simulink model "sim_2_twolink_joint_control_real"  (R2021a)
settings: Solver=ode45  StartTime=0.0  StopTime=15  MaxStep=0.01  RelTol=1e-5  EnableMultiTasking=on
values from neighbouring files (symbols this model uses):
  b1 = 0.01    [sim_params.m]    (also in sim_params_force.m)
  b2 = 0.01    [sim_params.m]    (also in sim_params_force.m)
  D = [zeros(n); eye(n)]    [control_comparison_script.m]    (also in gen_twolink_ss.m = reshape([0.0,0.0,0.0,0.0,0.0,0.0,0.0,0.0],[4,2]))
  D_T_Q = D'*Q    [control_comparison_script.m]
  epsilon = 0.1    [control_comparison_script.m]
  g = 9.80665    [sim_params.m]    (also in sim_params_force.m)
  joint_acc_variance = 0    [sim_params.m]    (also in sim_params_force.m)
  joint_pos_variance = joint_pos_precision^2    (= 0.0001)    [control_comparison_script.m]    (also in sim_params.m = 2.5e-05; sim_params_force.m = 2.5e-05)
  joint_vel_variance = 0    [sim_params.m]    (also in sim_params_force.m)
  Kd1 = 2.5    [control_comparison_script.m]
  Kd1_grav = 2.5    [control_comparison_script.m]
  Kd1_inv = 12    [control_comparison_script.m]
  Kd1_robust = 7    [control_comparison_script.m]
  Kd2 = 0.5    [control_comparison_script.m]
  Kd2_grav = 0.5    [control_comparison_script.m]
  Kd2_inv = 15    [control_comparison_script.m]
  Kd2_robust = 35    [control_comparison_script.m]
  Ki1 = 20    [control_comparison_script.m]
  Ki2 = 15    [control_comparison_script.m]
  Klqr = lqr(A,B,Q,R)    [control_comparison_script.m]
  Kp1 = 30    [control_comparison_script.m]
  Kp1_grav = 15    [control_comparison_script.m]
  Kp1_inv = 25    [control_comparison_script.m]
  Kp1_robust = 25    [control_comparison_script.m]
  Kp2 = 7    [control_comparison_script.m]
  Kp2_grav = 3.5    [control_comparison_script.m]
  Kp2_inv = 50    [control_comparison_script.m]
  Kp2_robust = 45    [control_comparison_script.m]
  Kpp = place(A,B,p)    [control_comparison_script.m]
  L1x = 0.3    [sim_params.m]    (also in sim_params_force.m)
  L1y = 0.050    (= 0.05)    [sim_params.m]    (also in sim_params_force.m)
  L1z = 0.05    [sim_params.m]    (also in sim_params_force.m)
  L2x = 0.15    [sim_params.m]    (also in sim_params_force.m = 0.3)
  L2y = 0.05    [sim_params.m]    (also in sim_params_force.m)
  L2z = 0.05    [sim_params.m]    (also in sim_params_force.m)
  length_dev = (100+randi([-param_dev,param_dev],1))/100.0    [control_comparison_script.m]
  m1 = m1*1.25    [control_comparison_script.m]    (also in sim_params.m = 2.775; sim_params_force.m = 2.775)
  m2 = m2*1.25    [control_comparison_script.m]    (also in sim_params.m = 1.3875; sim_params_force.m = 2.775)
  m_dev = (100+randi([-param_dev,param_dev],1))/100.0    [control_comparison_script.m]
  max_joint_torque1 = 20    [sim_params.m]    (also in sim_params_force.m)
  max_joint_torque2 = 10    [sim_params.m]    (also in sim_params_force.m = 20)
  N1 = 100    [control_comparison_script.m]
  N1_grav = 100    [control_comparison_script.m]
  N1_inv = 50    [control_comparison_script.m]
  N1_robust = 50    [control_comparison_script.m]
  N2 = 100    [control_comparison_script.m]
  N2_grav = 100    [control_comparison_script.m]
  N2_inv = 50    [control_comparison_script.m]
  N2_robust = 50    [control_comparison_script.m]
  rho = [1;1]    [control_comparison_script.m]
  theta1_0 = 0    [sim_params.m]    (also in sim_params_force.m = 1.57079632679)
  theta1_dot_0 = 0    [sim_params.m]    (also in sim_params_force.m)
  theta2_0 = 0    [sim_params.m]    (also in sim_params_force.m = -1.57079632679)
  theta2_dot_0 = 0    [sim_params.m]    (also in sim_params_force.m)
  Tsample = 0.001    [sim_params.m]    (also in sim_params_force.m)
  vis_dev = (100+randi([-param_dev,param_dev],1))/100.0    [control_comparison_script.m]
undefined symbols (not defined in the file or in its folder): gs, Ksm, phi_sm, sigbuilder_block, X, Y, Z
libraries: pid_lib x18, sm_lib x11, spsFirstOrderFilterLib x10, simulink_extras x10, nesl_utility x10, dspmtrx3 x2
(part 3 of 4)

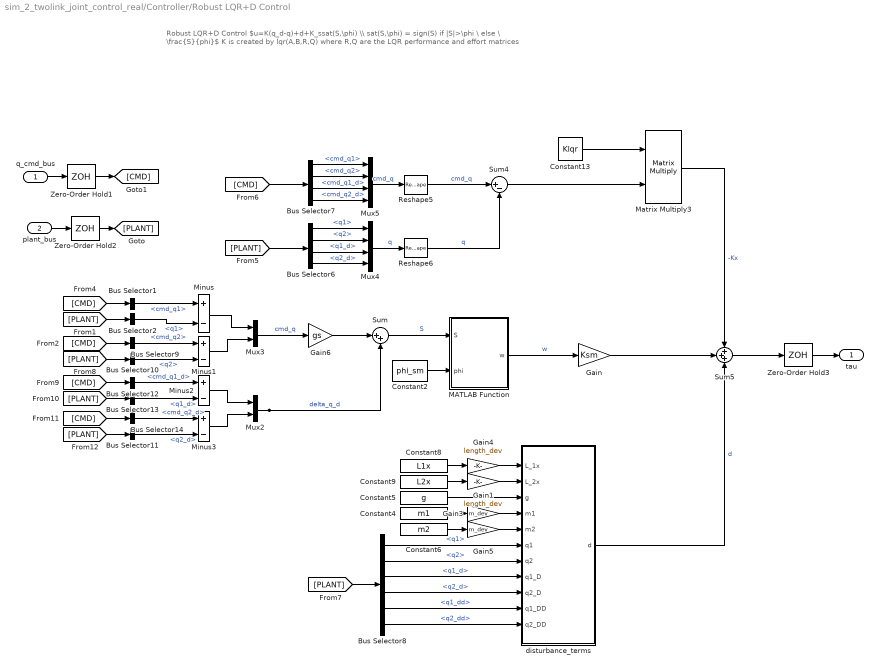
== system sim_2_twolink_joint_control_real/Controller/Robust LQR+D Control ==
  note: Robust LQR+D Control
      | $u=K(q_d-q)+d+K_ssat(S,\phi) \\ sat(S,\phi) = sign(S) if |S|>\phi \ else \ \frac{S}{phi}$
      | K is created by lqr(A,B,R,Q) where R,Q are the LQR performance and effort matrices
  q_cmd_bus : Inport
  plant_bus : Inport  Port=2
  Bus Selector1 : BusSelector  OutputSignals=cmd_q1
  Bus Selector10 : BusSelector  OutputSignals=q2
  Bus Selector11 : BusSelector  OutputSignals=q2_d
  Bus Selector12 : BusSelector  OutputSignals=cmd_q1_d
  Bus Selector13 : BusSelector  OutputSignals=q1_d
  Bus Selector14 : BusSelector  OutputSignals=cmd_q2_d
  Bus Selector2 : BusSelector  OutputSignals=q1
  Bus Selector6 : BusSelector  OutputSignals=q1,q2,q1_d,q2_d
  Bus Selector7 : BusSelector  OutputSignals=cmd_q1,cmd_q2,cmd_q1_d,cmd_q2_d
  Bus Selector8 : BusSelector  OutputSignals=q1,q2,q1_d,q2_d,q1_dd,q2_dd
  Bus Selector9 : BusSelector  OutputSignals=cmd_q2
  Constant13 : Constant  Value=Klqr  VectorParams1D=off
  Constant2 : Constant  Value=phi_sm
  Constant4 : Constant  Value=m1
  Constant5 : Constant  Value=g
  Constant6 : Constant  Value=m2
  Constant8 : Constant  Value=L1x
  Constant9 : Constant  Value=L2x
  Gain : Gain  Gain=Ksm
  Gain1 : Gain  Gain=length_dev
  Gain3 : Gain  Gain=m_dev
  Gain4 : Gain  Gain=length_dev
  Gain5 : Gain  Gain=m_dev
  Gain6 : Gain  Gain=gs
  MATLAB Function : MATLAB Function  TreatAsAtomicUnit=on
  Matrix Multiply3 : Product  Multiplication=Matrix(*)
  Minus{,1..3} (4 alike) : Sum  Inputs=+-
  Mux2 : Mux  Inputs=2
  Mux3 : Mux  Inputs=2
  Mux4 : Mux
  Mux5 : Mux
  Reshape5 : Reshape  OutputDimensionality=Column vector (2-D)
  Reshape6 : Reshape  OutputDimensionality=Column vector (2-D)
  Sum : Sum  Inputs=|++
  Sum4 : Sum  Inputs=|+-
  Sum5 : Sum  Inputs=+++
  Zero-Order Hold1 : ZeroOrderHold  SampleTime=0.001
  Zero-Order Hold2 : ZeroOrderHold  SampleTime=0.001
  Zero-Order Hold3 : ZeroOrderHold  SampleTime=0.001
  disturbance_terms : MATLAB Function  TreatAsAtomicUnit=on
  tau : Outport
  wires:
  plant_bus/1 -> Zero-Order Hold2/1
  q_cmd_bus/1 -> Zero-Order Hold1/1
  Zero-Order Hold1/1 -> [CMD]
  Zero-Order Hold2/1 -> [PLANT]
  Zero-Order Hold3/1 -> tau/1
  Constant4/1 -> Gain3/1
  Bus Selector6/1 -> Mux4/1  "<q1>"
  Bus Selector7/4 -> Mux5/4  "<cmd_q2_d>"
  Mux4/1 -> Reshape6/1  "q"
  Bus Selector7/2 -> Mux5/2  "<cmd_q2>"
  [PLANT] -> Bus Selector6/1
  Mux5/1 -> Reshape5/1  "cmd_q"
  Bus Selector6/2 -> Mux4/2  "<q2>"
  Bus Selector6/4 -> Mux4/4  "<q2_d>"
  Matrix Multiply3/1 -> Sum5/1  "-Kx"
  Bus Selector6/3 -> Mux4/3  "<q1_d>"
  Reshape5/1 -> Sum4/1  "cmd_q"
  Sum4/1 -> Matrix Multiply3/2
  Gain5/1 -> disturbance_terms/5(m2)
  [CMD] -> Bus Selector7/1
  Constant13/1 -> Matrix Multiply3/1
  Gain3/1 -> disturbance_terms/4(m1)
  Bus Selector7/3 -> Mux5/3  "<cmd_q1_d>"
  Reshape6/1 -> Sum4/2  "q"
  Bus Selector7/1 -> Mux5/1  "<cmd_q1>"
  Bus Selector8/5 -> disturbance_terms/10(q1_DD)  "<q1_dd>"
  disturbance_terms/1(d) -> Sum5/3  "d"
  Bus Selector8/3 -> disturbance_terms/8(q1_D)  "<q1_d>"
  Gain1/1 -> disturbance_terms/2(L_2x)
  Bus Selector8/6 -> disturbance_terms/11(q2_DD)  "<q2_dd>"
  Bus Selector8/4 -> disturbance_terms/9(q2_D)  "<q2_d>"
  Constant5/1 -> disturbance_terms/3(g)
  Constant8/1 -> Gain4/1
  Sum5/1 -> Zero-Order Hold3/1
  Bus Selector8/2 -> disturbance_terms/7(q2)  "<q2>"
  Constant9/1 -> Gain1/1
  Gain4/1 -> disturbance_terms/1(L_1x)
  [PLANT] -> Bus Selector8/1
  Bus Selector8/1 -> disturbance_terms/6(q1)  "<q1>"
  Constant6/1 -> Gain5/1
  Constant2/1 -> MATLAB Function/2(phi)
  [CMD] -> Bus Selector12/1
  Bus Selector1/1 -> Minus/1  "<cmd_q1>"
  [PLANT] -> Bus Selector13/1
  [PLANT] -> Bus Selector10/1
  [CMD] -> Bus Selector1/1
  Minus/1 -> Mux3/1
  [PLANT] -> Bus Selector11/1
  Minus3/1 -> Mux2/2
  [CMD] -> Bus Selector9/1
  Bus Selector12/1 -> Minus2/1  "<cmd_q1_d>"
  Bus Selector10/1 -> Minus1/2  "<q2>"
  Bus Selector2/1 -> Minus/2  "<q1>"
  Bus Selector9/1 -> Minus1/1  "<cmd_q2>"
  [PLANT] -> Bus Selector2/1
  Bus Selector11/1 -> Minus3/2  "<q2_d>"
  Bus Selector13/1 -> Minus2/2  "<q1_d>"
  Bus Selector14/1 -> Minus3/1  "<cmd_q2_d>"
  Minus2/1 -> Mux2/1
  [CMD] -> Bus Selector14/1
  Minus1/1 -> Mux3/2
  Sum/1 -> MATLAB Function/1(S)  "S"
  MATLAB Function/1(w) -> Gain/1  "w"
  Gain/1 -> Sum5/2
  Mux3/1 -> Gain6/1  "cmd_q"
  Mux2/1 -> Sum/2  "delta_q_d"
  Gain6/1 -> Sum/1

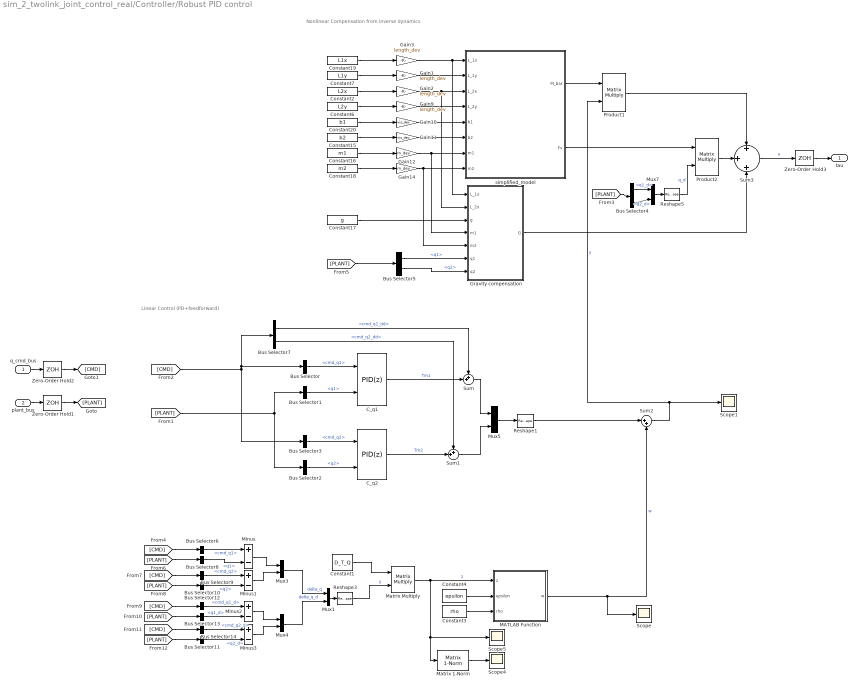
== system sim_2_twolink_joint_control_real/Controller/Robust PID control  ==
  note: Nonlinear Compensation from inverse dynamics
  note: Linear Control (PD+feedforward)
  q_cmd_bus : Inport
  plant_bus : Inport  Port=2
  Bus Selector : BusSelector  OutputSignals=cmd_q1
  Bus Selector1 : BusSelector  OutputSignals=q1
  Bus Selector10 : BusSelector  OutputSignals=q2
  Bus Selector11 : BusSelector  OutputSignals=q2_d
  Bus Selector12 : BusSelector  OutputSignals=cmd_q1_d
  Bus Selector13 : BusSelector  OutputSignals=q1_d
  Bus Selector14 : BusSelector  OutputSignals=cmd_q2_d
  Bus Selector2 : BusSelector  OutputSignals=q2
  Bus Selector3 : BusSelector  OutputSignals=cmd_q2
  Bus Selector4 : BusSelector  OutputSignals=q1_d,q2_d
  Bus Selector5 : BusSelector  OutputSignals=q1,q2
  Bus Selector6 : BusSelector  OutputSignals=cmd_q1
  Bus Selector7 : BusSelector  OutputSignals=cmd_q1_dd,cmd_q2_dd
  Bus Selector8 : BusSelector  OutputSignals=q1
  Bus Selector9 : BusSelector  OutputSignals=cmd_q2
  C_q1 : pid_lib/PID Controller (2DOF)  Controller=PID  Form=Parallel  TimeDomain=Discrete-time  UseExternalTs=off  SampleTime=Tsample  IntegratorMethod=Forward Euler  FilterMethod=Forward Euler  ControllerParametersSource=internal  P=30  I=20  D=15  UseFilter=on  N=50  b=1  c=1  TunerSelectOption=Transfer Function Based (PID Tuner App)  InitialConditionSource=internal  InitialConditionForIntegrator=0  InitialConditionForFilter=0  DifferentiatorICPrevScaledInput=0  ExternalReset=none  TrackingMode=off  Kt=1  LimitOutput=off  SatLimitsSource=internal  UpperSaturationLimit=inf  LowerSaturationLimit=-inf  LinearizeAsGain=on  AntiWindupMode=none  Kb=1  POutMin=[]  POutMax=[]  IOutMin=[]  IOutMax=[]  DOutMin=[]  DOutMax=[]  NOutMin=[]  NOutMax=[]  bOutMin=[]  bOutMax=[]  cOutMin=[]  cOutMax=[]  SumOutMin=[]  SumOutMax=[]  SaturationOutMin=[]  SaturationOutMax=[]  PParamMin=[]  PParamMax=[]  IParamMin=[]  IParamMax=[]  DParamMin=[]  DParamMax=[]  NParamMin=[]  NParamMax=[]  bParamMin=[]  bParamMax=[]  cParamMin=[]  cParamMax=[]  KbParamMin=[]  KbParamMax=[]  KtParamMin=[]  KtParamMax=[]  KbOutMin=[]  KbOutMax=[]  KtOutMin=[]  KtOutMax=[]  IntegratorOutMin=[]  IntegratorOutMax=[]  FilterOutMin=[]  FilterOutMax=[]  SumI1OutMin=[]  SumI1OutMax=[]  SumI2OutMin=[]  SumI2OutMax=[]  SumI3OutMin=[]  SumI3OutMax=[]  SumI4OutMin=[]  SumI4OutMax=[]  SumDOutMin=[]  SumDOutMax=[]  Sum1OutMin=[]  Sum1OutMax=[]  Sum2OutMin=[]  Sum2OutMax=[]  Sum3OutMin=[]  Sum3OutMax=[]  DifferentiatorOutMin=[]  DifferentiatorOutMax=[]  FilterDiffOutCoefMin=[]  FilterDiffOutCoefMax=[]  ReciprocalOutMin=[]  ReciprocalOutMax=[]  SumDenOutMin=[]  SumDenOutMax=[]  SumNumOutMin=[]  SumNumOutMax=[]  DivideOutMin=[]  DivideOutMax=[]  UdiffTsProdOutMin=[]  UdiffTsProdOutMax=[]  NTsProdOutMin=[]  NTsProdOutMax=[]  UintegralTsProdOutMin=[]  UintegralTsProdOutMax=[]  UngainTsProdOutMin=[]  UngainTsProdOutMax=[]  IntegratorContinuousStateAttributes=''  IntegratorStateMustResolveToSignalObject=off  IntegratorRTWStateStorageClass=Auto  FilterContinuousStateAttributes=''  FilterStateMustResolveToSignalObject=off  FilterRTWStateStorageClass=Auto  ParallelPVariant=InternalParameters  IdealPVariant=Disabled  IVariant=InternalParameters  DVariant=InternalParameters  bVariant=InternalParameters  cVariant=InternalParameters  IntegratorVariant=Discrete  SatVariant=Disabled  AWVariant=Passthrough  PCopyVariant=Disabled  TRVariant=Disabled  FdbkBlocksVariant=Forward  IdealPFdbkVariant=Disabled  SatFdbkVariant=Disabled  DerivativeFilterVariant=ForwardEulerFilter  NVariant=InternalParameters  NCopyVariant=Disabled  FilterICVariant=InternalICsFilter  IntegratorICVariant=InternalICs  ExternalResetVariant=Disabled  TRSumVariant=Passthrough  SumFdbkVariant=Disabled  SumVariant=Sum_PID  TsampFilterVariant=InternalTs  TsampNgainVariant=Passthrough  TsampIntegralVariant=Passthrough  ExternalSaturationOutDataTypeStr=Inherit: Same as second input
      settings: SourceProductBaseCode=SL
  C_q2 : pid_lib/PID Controller (2DOF)  Controller=PID  Form=Parallel  TimeDomain=Discrete-time  UseExternalTs=off  SampleTime=Tsample  IntegratorMethod=Forward Euler  FilterMethod=Forward Euler  ControllerParametersSource=internal  P=100  I=30  D=50  UseFilter=on  N=50  b=1  c=1  TunerSelectOption=Transfer Function Based (PID Tuner App)  InitialConditionSource=internal  InitialConditionForIntegrator=0  InitialConditionForFilter=0  DifferentiatorICPrevScaledInput=0  ExternalReset=none  TrackingMode=off  Kt=1  LimitOutput=off  SatLimitsSource=internal  UpperSaturationLimit=inf  LowerSaturationLimit=-inf  LinearizeAsGain=on  AntiWindupMode=none  Kb=1  POutMin=[]  POutMax=[]  IOutMin=[]  IOutMax=[]  DOutMin=[]  DOutMax=[]  NOutMin=[]  NOutMax=[]  bOutMin=[]  bOutMax=[]  cOutMin=[]  cOutMax=[]  SumOutMin=[]  SumOutMax=[]  SaturationOutMin=[]  SaturationOutMax=[]  PParamMin=[]  PParamMax=[]  IParamMin=[]  IParamMax=[]  DParamMin=[]  DParamMax=[]  NParamMin=[]  NParamMax=[]  bParamMin=[]  bParamMax=[]  cParamMin=[]  cParamMax=[]  KbParamMin=[]  KbParamMax=[]  KtParamMin=[]  KtParamMax=[]  KbOutMin=[]  KbOutMax=[]  KtOutMin=[]  KtOutMax=[]  IntegratorOutMin=[]  IntegratorOutMax=[]  FilterOutMin=[]  FilterOutMax=[]  SumI1OutMin=[]  SumI1OutMax=[]  SumI2OutMin=[]  SumI2OutMax=[]  SumI3OutMin=[]  SumI3OutMax=[]  SumI4OutMin=[]  SumI4OutMax=[]  SumDOutMin=[]  SumDOutMax=[]  Sum1OutMin=[]  Sum1OutMax=[]  Sum2OutMin=[]  Sum2OutMax=[]  Sum3OutMin=[]  Sum3OutMax=[]  DifferentiatorOutMin=[]  DifferentiatorOutMax=[]  FilterDiffOutCoefMin=[]  FilterDiffOutCoefMax=[]  ReciprocalOutMin=[]  ReciprocalOutMax=[]  SumDenOutMin=[]  SumDenOutMax=[]  SumNumOutMin=[]  SumNumOutMax=[]  DivideOutMin=[]  DivideOutMax=[]  UdiffTsProdOutMin=[]  UdiffTsProdOutMax=[]  NTsProdOutMin=[]  NTsProdOutMax=[]  UintegralTsProdOutMin=[]  UintegralTsProdOutMax=[]  UngainTsProdOutMin=[]  UngainTsProdOutMax=[]  IntegratorContinuousStateAttributes=''  IntegratorStateMustResolveToSignalObject=off  IntegratorRTWStateStorageClass=Auto  FilterContinuousStateAttributes=''  FilterStateMustResolveToSignalObject=off  FilterRTWStateStorageClass=Auto  ParallelPVariant=InternalParameters  IdealPVariant=Disabled  IVariant=InternalParameters  DVariant=InternalParameters  bVariant=InternalParameters  cVariant=InternalParameters  IntegratorVariant=Discrete  SatVariant=Disabled  AWVariant=Passthrough  PCopyVariant=Disabled  TRVariant=Disabled  FdbkBlocksVariant=Forward  IdealPFdbkVariant=Disabled  SatFdbkVariant=Disabled  DerivativeFilterVariant=ForwardEulerFilter  NVariant=InternalParameters  NCopyVariant=Disabled  FilterICVariant=InternalICsFilter  IntegratorICVariant=InternalICs  ExternalResetVariant=Disabled  TRSumVariant=Passthrough  SumFdbkVariant=Disabled  SumVariant=Sum_PID  TsampFilterVariant=InternalTs  TsampNgainVariant=Passthrough  TsampIntegralVariant=Passthrough  ExternalSaturationOutDataTypeStr=Inherit: Same as second input
      settings: SourceProductBaseCode=SL
  Constant1 : Constant  Value=D_T_Q
  Constant15 : Constant  Value=b2
  Constant16 : Constant  Value=m1
  Constant17 : Constant  Value=g
  Constant18 : Constant  Value=m2
  Constant19 : Constant  Value=L1x
  Constant2 : Constant  Value=L2x
  Constant20 : Constant  Value=b1
  Constant3 : Constant  Value=rho
  Constant4 : Constant  Value=epsilon
  Constant6 : Constant  Value=L2y
  Constant7 : Constant  Value=L1y
  Gain{1..3,9} (4 alike) : Gain  Gain=length_dev
  Gain10 : Gain  Gain=vis_dev
  Gain11 : Gain  Gain=vis_dev
  Gain12 : Gain  Gain=m_dev
  Gain14 : Gain  Gain=m_dev
  Gravity compensation : MATLAB Function  TreatAsAtomicUnit=on
  MATLAB Function : MATLAB Function  TreatAsAtomicUnit=on
  Matrix 1-Norm : dspmtrx3/Matrix  1-Norm  roundingMode=Floor  overflowMode=off  outputDataTypeStr=Inherit: Same as accumulator  outputMin=[]  outputMax=[]  outputLastDataTypeStr=Inherit: Same as accumulator
      settings: SourceProductBaseCode=DS
  Matrix Multiply : Product  Multiplication=Matrix(*)
  Minus{,1..3} (4 alike) : Sum  Inputs=+-
  Mux{1,3..5,7} (5 alike) : Mux  Inputs=2
  Product1 : Product  Multiplication=Matrix(*)
  Product2 : Product  Multiplication=Matrix(*)
  Reshape1 : Reshape  OutputDimensionality=Column vector (2-D)
  Reshape3 : Reshape  OutputDimensionality=Column vector (2-D)
  Reshape5 : Reshape  OutputDimensionality=Column vector (2-D)
  Scope{,1,4..5} (4 alike) : Scope
  Sum : Sum  Inputs=++|
  Sum1 : Sum  Inputs=++|
  Sum2 : Sum  Inputs=|++
  Sum3 : Sum  Inputs=+|+|+
  Zero-Order Hold1 : ZeroOrderHold  SampleTime=0.001
  Zero-Order Hold2 : ZeroOrderHold  SampleTime=0.001
  Zero-Order Hold3 : ZeroOrderHold  SampleTime=0.001
  simplified_model : MATLAB Function  TreatAsAtomicUnit=on
  tau : Outport
  wires:
  C_q1/1 -> Sum/2  "Tm1"
  q_cmd_bus/1 -> Zero-Order Hold2/1
  plant_bus/1 -> Zero-Order Hold1/1
  Bus Selector2/1 -> C_q2/2  "<q2>"
  Bus Selector3/1 -> C_q2/1  "<cmd_q2>"
  Bus Selector1/1 -> C_q1/2  "<q1>"
  Bus Selector/1 -> C_q1/1  "<cmd_q1>"
  [PLANT] -> Bus Selector1/1, Bus Selector2/1
  Constant16/1 -> Gain12/1
  Constant20/1 -> Gain10/1
  Constant2/1 -> Gain2/1
  Bus Selector5/1 -> Gravity compensation/6(q1)  "<q1>"
  Constant19/1 -> Gain3/1
  Constant15/1 -> Gain11/1
  Constant6/1 -> Gain9/1
  Constant7/1 -> Gain1/1
  Constant18/1 -> Gain14/1
  [PLANT] -> Bus Selector5/1
  Bus Selector5/2 -> Gravity compensation/7(q2)  "<q2>"
  Mux5/1 -> Reshape1/1
  Sum3/1 -> Zero-Order Hold3/1  "u"
  [CMD] -> Bus Selector7/1, Bus Selector/1, Bus Selector3/1
  Bus Selector7/2 -> Sum1/1  "<cmd_q2_dd>"
  Sum/1 -> Mux5/1
  C_q2/1 -> Sum1/2  "Tm2"
  Sum1/1 -> Mux5/2
  [PLANT] -> Bus Selector4/1
  Bus Selector4/1 -> Mux7/1  "<q1_d>"
  Bus Selector4/2 -> Mux7/2  "<q2_d>"
  Mux7/1 -> Reshape5/1
  Reshape5/1 -> Product2/2  "q_d"
  Sum2/1 -> Scope1/1, Product1/2  "y"
  Bus Selector7/1 -> Sum/1  "<cmd_q1_dd>"
  Gain1/1 -> simplified_model/2(L_1y)
  Gain2/1 -> Gravity compensation/2(L_2x), simplified_model/3(L_2x)
  Gain9/1 -> simplified_model/4(L_2y)
  Gain10/1 -> simplified_model/5(b1)
  Gain11/1 -> simplified_model/6(b2)
  Gain12/1 -> Gravity compensation/4(m1), simplified_model/7(m1)
  Gain14/1 -> Gravity compensation/5(m2), simplified_model/8(m2)
  Bus Selector6/1 -> Minus/1  "<cmd_q1>"
  Bus Selector8/1 -> Minus/2  "<q1>"
  [CMD] -> Bus Selector6/1
  [PLANT] -> Bus Selector8/1
  [PLANT] -> Bus Selector10/1
  Bus Selector9/1 -> Minus1/1  "<cmd_q2>"
  Bus Selector10/1 -> Minus1/2  "<q2>"
  [CMD] -> Bus Selector9/1
  Bus Selector13/1 -> Minus2/2  "<q1_d>"
  [CMD] -> Bus Selector12/1
  Bus Selector11/1 -> Minus3/2  "<q2_d>"
  Bus Selector12/1 -> Minus2/1  "<cmd_q1_d>"
  [CMD] -> Bus Selector14/1
  Bus Selector14/1 -> Minus3/1  "<cmd_q2_d>"
  [PLANT] -> Bus Selector13/1
  [PLANT] -> Bus Selector11/1
  Mux1/1 -> Reshape3/1
  Minus/1 -> Mux3/1
  Minus1/1 -> Mux3/2
  Mux3/1 -> Mux1/1  "delta_q"
  Minus3/1 -> Mux4/2
  Minus2/1 -> Mux4/1
  Mux4/1 -> Mux1/2  "delta_q_d"
  Reshape3/1 -> Matrix Multiply/2  "y"
  Constant1/1 -> Matrix Multiply/1
  Matrix Multiply/1 -> Scope5/1, Matrix 1-Norm/1, MATLAB Function/1(z)  "z"
  MATLAB Function/1(w) -> Sum2/2, Scope/1  "w"
  Reshape1/1 -> Sum2/1
  Constant4/1 -> MATLAB Function/2(epsilon)
  Constant3/1 -> MATLAB Function/3(rho)
  Matrix 1-Norm/1 -> Scope4/1
  Zero-Order Hold2/1 -> [CMD]
  Zero-Order Hold1/1 -> [PLANT]
  Zero-Order Hold3/1 -> tau/1
  Constant17/1 -> Gravity compensation/3(g)
  Gain3/1 -> Gravity compensation/1(L_1x), simplified_model/1(L_1x)
  simplified_model/1(M_bar) -> Product1/1
  Product2/1 -> Sum3/2
  Product1/1 -> Sum3/1
  simplified_model/2(Fv) -> Product2/1
  Gravity compensation/1(G) -> Sum3/3

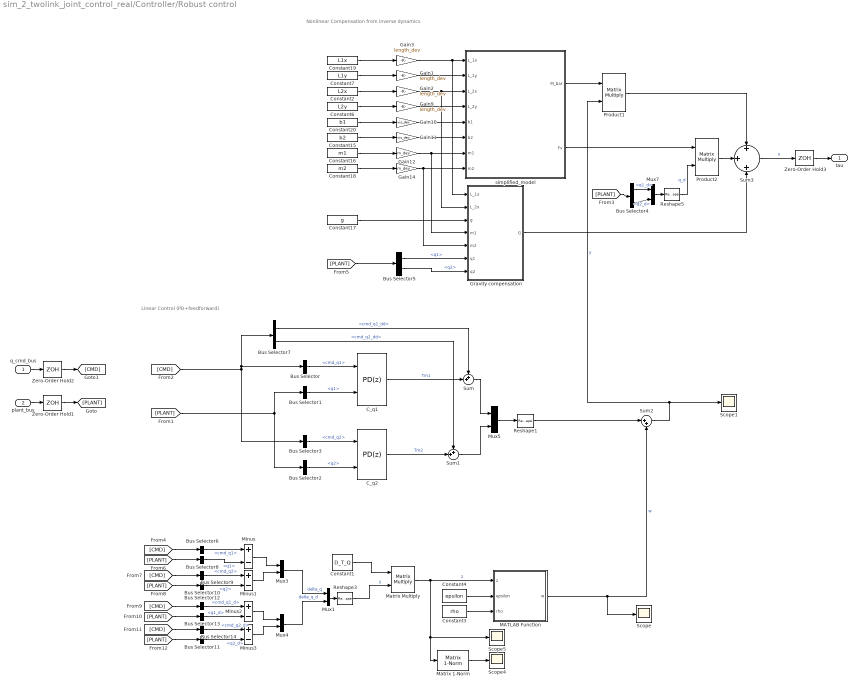
== system sim_2_twolink_joint_control_real/Controller/Robust control  ==
  note: Nonlinear Compensation from inverse dynamics
  note: Linear Control (PD+feedforward)
  q_cmd_bus : Inport
  plant_bus : Inport  Port=2
  Bus Selector : BusSelector  OutputSignals=cmd_q1
  Bus Selector1 : BusSelector  OutputSignals=q1
  Bus Selector10 : BusSelector  OutputSignals=q2
  Bus Selector11 : BusSelector  OutputSignals=q2_d
  Bus Selector12 : BusSelector  OutputSignals=cmd_q1_d
  Bus Selector13 : BusSelector  OutputSignals=q1_d
  Bus Selector14 : BusSelector  OutputSignals=cmd_q2_d
  Bus Selector2 : BusSelector  OutputSignals=q2
  Bus Selector3 : BusSelector  OutputSignals=cmd_q2
  Bus Selector4 : BusSelector  OutputSignals=q1_d,q2_d
  Bus Selector5 : BusSelector  OutputSignals=q1,q2
  Bus Selector6 : BusSelector  OutputSignals=cmd_q1
  Bus Selector7 : BusSelector  OutputSignals=cmd_q1_dd,cmd_q2_dd
  Bus Selector8 : BusSelector  OutputSignals=q1
  Bus Selector9 : BusSelector  OutputSignals=cmd_q2
  C_q1 : pid_lib/PID Controller (2DOF)  Controller=PD  Form=Parallel  TimeDomain=Discrete-time  UseExternalTs=off  SampleTime=Tsample  IntegratorMethod=Forward Euler  FilterMethod=Forward Euler  ControllerParametersSource=internal  P=Kp1_robust  I=Kd1_robust  D=Kd1_robust  UseFilter=on  N=N1_robust  b=1  c=1  TunerSelectOption=Transfer Function Based (PID Tuner App)  InitialConditionSource=internal  InitialConditionForIntegrator=0  InitialConditionForFilter=0  DifferentiatorICPrevScaledInput=0  ExternalReset=none  TrackingMode=off  Kt=1  LimitOutput=off  SatLimitsSource=internal  UpperSaturationLimit=inf  LowerSaturationLimit=-inf  LinearizeAsGain=on  AntiWindupMode=none  Kb=1  POutMin=[]  POutMax=[]  IOutMin=[]  IOutMax=[]  DOutMin=[]  DOutMax=[]  NOutMin=[]  NOutMax=[]  bOutMin=[]  bOutMax=[]  cOutMin=[]  cOutMax=[]  SumOutMin=[]  SumOutMax=[]  SaturationOutMin=[]  SaturationOutMax=[]  PParamMin=[]  PParamMax=[]  IParamMin=[]  IParamMax=[]  DParamMin=[]  DParamMax=[]  NParamMin=[]  NParamMax=[]  bParamMin=[]  bParamMax=[]  cParamMin=[]  cParamMax=[]  KbParamMin=[]  KbParamMax=[]  KtParamMin=[]  KtParamMax=[]  KbOutMin=[]  KbOutMax=[]  KtOutMin=[]  KtOutMax=[]  IntegratorOutMin=[]  IntegratorOutMax=[]  FilterOutMin=[]  FilterOutMax=[]  SumI1OutMin=[]  SumI1OutMax=[]  SumI2OutMin=[]  SumI2OutMax=[]  SumI3OutMin=[]  SumI3OutMax=[]  SumI4OutMin=[]  SumI4OutMax=[]  SumDOutMin=[]  SumDOutMax=[]  Sum1OutMin=[]  Sum1OutMax=[]  Sum2OutMin=[]  Sum2OutMax=[]  Sum3OutMin=[]  Sum3OutMax=[]  DifferentiatorOutMin=[]  DifferentiatorOutMax=[]  FilterDiffOutCoefMin=[]  FilterDiffOutCoefMax=[]  ReciprocalOutMin=[]  ReciprocalOutMax=[]  SumDenOutMin=[]  SumDenOutMax=[]  SumNumOutMin=[]  SumNumOutMax=[]  DivideOutMin=[]  DivideOutMax=[]  UdiffTsProdOutMin=[]  UdiffTsProdOutMax=[]  NTsProdOutMin=[]  NTsProdOutMax=[]  UintegralTsProdOutMin=[]  UintegralTsProdOutMax=[]  UngainTsProdOutMin=[]  UngainTsProdOutMax=[]  IntegratorContinuousStateAttributes=''  IntegratorStateMustResolveToSignalObject=off  IntegratorRTWStateStorageClass=Auto  FilterContinuousStateAttributes=''  FilterStateMustResolveToSignalObject=off  FilterRTWStateStorageClass=Auto  ParallelPVariant=InternalParameters  IdealPVariant=Disabled  IVariant=Disabled  DVariant=InternalParameters  bVariant=InternalParameters  cVariant=InternalParameters  IntegratorVariant=Disabled  SatVariant=Disabled  AWVariant=Disabled  PCopyVariant=Disabled  TRVariant=Disabled  FdbkBlocksVariant=Forward  IdealPFdbkVariant=Disabled  SatFdbkVariant=Disabled  DerivativeFilterVariant=ForwardEulerFilter  NVariant=InternalParameters  NCopyVariant=Disabled  FilterICVariant=InternalICsFilter  IntegratorICVariant=Disabled  ExternalResetVariant=Disabled  TRSumVariant=Passthrough  SumFdbkVariant=Disabled  SumVariant=Sum_PD  TsampFilterVariant=InternalTs  TsampNgainVariant=Passthrough  TsampIntegralVariant=Disabled_SignalSpec  ExternalSaturationOutDataTypeStr=Inherit: Same as second input
      settings: SourceProductBaseCode=SL
  C_q2 : pid_lib/PID Controller (2DOF)  Controller=PD  Form=Parallel  TimeDomain=Discrete-time  UseExternalTs=off  SampleTime=Tsample  IntegratorMethod=Forward Euler  FilterMethod=Forward Euler  ControllerParametersSource=internal  P=Kp2_robust  I=Kd2_robust  D=Kd2_robust  UseFilter=on  N=N2_robust  b=1  c=1  TunerSelectOption=Transfer Function Based (PID Tuner App)  InitialConditionSource=internal  InitialConditionForIntegrator=0  InitialConditionForFilter=0  DifferentiatorICPrevScaledInput=0  ExternalReset=none  TrackingMode=off  Kt=1  LimitOutput=off  SatLimitsSource=internal  UpperSaturationLimit=inf  LowerSaturationLimit=-inf  LinearizeAsGain=on  AntiWindupMode=none  Kb=1  POutMin=[]  POutMax=[]  IOutMin=[]  IOutMax=[]  DOutMin=[]  DOutMax=[]  NOutMin=[]  NOutMax=[]  bOutMin=[]  bOutMax=[]  cOutMin=[]  cOutMax=[]  SumOutMin=[]  SumOutMax=[]  SaturationOutMin=[]  SaturationOutMax=[]  PParamMin=[]  PParamMax=[]  IParamMin=[]  IParamMax=[]  DParamMin=[]  DParamMax=[]  NParamMin=[]  NParamMax=[]  bParamMin=[]  bParamMax=[]  cParamMin=[]  cParamMax=[]  KbParamMin=[]  KbParamMax=[]  KtParamMin=[]  KtParamMax=[]  KbOutMin=[]  KbOutMax=[]  KtOutMin=[]  KtOutMax=[]  IntegratorOutMin=[]  IntegratorOutMax=[]  FilterOutMin=[]  FilterOutMax=[]  SumI1OutMin=[]  SumI1OutMax=[]  SumI2OutMin=[]  SumI2OutMax=[]  SumI3OutMin=[]  SumI3OutMax=[]  SumI4OutMin=[]  SumI4OutMax=[]  SumDOutMin=[]  SumDOutMax=[]  Sum1OutMin=[]  Sum1OutMax=[]  Sum2OutMin=[]  Sum2OutMax=[]  Sum3OutMin=[]  Sum3OutMax=[]  DifferentiatorOutMin=[]  DifferentiatorOutMax=[]  FilterDiffOutCoefMin=[]  FilterDiffOutCoefMax=[]  ReciprocalOutMin=[]  ReciprocalOutMax=[]  SumDenOutMin=[]  SumDenOutMax=[]  SumNumOutMin=[]  SumNumOutMax=[]  DivideOutMin=[]  DivideOutMax=[]  UdiffTsProdOutMin=[]  UdiffTsProdOutMax=[]  NTsProdOutMin=[]  NTsProdOutMax=[]  UintegralTsProdOutMin=[]  UintegralTsProdOutMax=[]  UngainTsProdOutMin=[]  UngainTsProdOutMax=[]  IntegratorContinuousStateAttributes=''  IntegratorStateMustResolveToSignalObject=off  IntegratorRTWStateStorageClass=Auto  FilterContinuousStateAttributes=''  FilterStateMustResolveToSignalObject=off  FilterRTWStateStorageClass=Auto  ParallelPVariant=InternalParameters  IdealPVariant=Disabled  IVariant=Disabled  DVariant=InternalParameters  bVariant=InternalParameters  cVariant=InternalParameters  IntegratorVariant=Disabled  SatVariant=Disabled  AWVariant=Disabled  PCopyVariant=Disabled  TRVariant=Disabled  FdbkBlocksVariant=Forward  IdealPFdbkVariant=Disabled  SatFdbkVariant=Disabled  DerivativeFilterVariant=ForwardEulerFilter  NVariant=InternalParameters  NCopyVariant=Disabled  FilterICVariant=InternalICsFilter  IntegratorICVariant=Disabled  ExternalResetVariant=Disabled  TRSumVariant=Passthrough  SumFdbkVariant=Disabled  SumVariant=Sum_PD  TsampFilterVariant=InternalTs  TsampNgainVariant=Passthrough  TsampIntegralVariant=Disabled_SignalSpec  ExternalSaturationOutDataTypeStr=Inherit: Same as second input
      settings: SourceProductBaseCode=SL
  Constant1 : Constant  Value=D_T_Q
  Constant15 : Constant  Value=b2
  Constant16 : Constant  Value=m1
  Constant17 : Constant  Value=g
  Constant18 : Constant  Value=m2
  Constant19 : Constant  Value=L1x
  Constant2 : Constant  Value=L2x
  Constant20 : Constant  Value=b1
  Constant3 : Constant  Value=rho
  Constant4 : Constant  Value=epsilon
  Constant6 : Constant  Value=L2y
  Constant7 : Constant  Value=L1y
  Gain{1..3,9} (4 alike) : Gain  Gain=length_dev
  Gain10 : Gain  Gain=vis_dev
  Gain11 : Gain  Gain=vis_dev
  Gain12 : Gain  Gain=m_dev
  Gain14 : Gain  Gain=m_dev
  Gravity compensation : MATLAB Function  TreatAsAtomicUnit=on
  MATLAB Function : MATLAB Function  TreatAsAtomicUnit=on
  Matrix 1-Norm : dspmtrx3/Matrix  1-Norm  roundingMode=Floor  overflowMode=off  outputDataTypeStr=Inherit: Same as accumulator  outputMin=[]  outputMax=[]  outputLastDataTypeStr=Inherit: Same as accumulator
      settings: SourceProductBaseCode=DS
  Matrix Multiply : Product  Multiplication=Matrix(*)
  Minus{,1..3} (4 alike) : Sum  Inputs=+-
  Mux{1,3..5,7} (5 alike) : Mux  Inputs=2
  Product1 : Product  Multiplication=Matrix(*)
  Product2 : Product  Multiplication=Matrix(*)
  Reshape1 : Reshape  OutputDimensionality=Column vector (2-D)
  Reshape3 : Reshape  OutputDimensionality=Column vector (2-D)
  Reshape5 : Reshape  OutputDimensionality=Column vector (2-D)
  Scope{,1,4..5} (4 alike) : Scope
  Sum : Sum  Inputs=++|
  Sum1 : Sum  Inputs=++|
  Sum2 : Sum  Inputs=|++
  Sum3 : Sum  Inputs=+|+|+
  Zero-Order Hold1 : ZeroOrderHold  SampleTime=0.001
  Zero-Order Hold2 : ZeroOrderHold  SampleTime=0.001
  Zero-Order Hold3 : ZeroOrderHold  SampleTime=0.001
  simplified_model : MATLAB Function  TreatAsAtomicUnit=on
  tau : Outport
  wires:
  C_q1/1 -> Sum/2  "Tm1"
  q_cmd_bus/1 -> Zero-Order Hold2/1
  plant_bus/1 -> Zero-Order Hold1/1
  Bus Selector2/1 -> C_q2/2  "<q2>"
  Bus Selector3/1 -> C_q2/1  "<cmd_q2>"
  Bus Selector1/1 -> C_q1/2  "<q1>"
  Bus Selector/1 -> C_q1/1  "<cmd_q1>"
  [PLANT] -> Bus Selector1/1, Bus Selector2/1
  Constant16/1 -> Gain12/1
  Constant20/1 -> Gain10/1
  Constant2/1 -> Gain2/1
  Bus Selector5/1 -> Gravity compensation/6(q1)  "<q1>"
  Constant19/1 -> Gain3/1
  Constant15/1 -> Gain11/1
  Constant6/1 -> Gain9/1
  Constant7/1 -> Gain1/1
  Constant18/1 -> Gain14/1
  [PLANT] -> Bus Selector5/1
  Bus Selector5/2 -> Gravity compensation/7(q2)  "<q2>"
  Mux5/1 -> Reshape1/1
  Sum3/1 -> Zero-Order Hold3/1  "u"
  [CMD] -> Bus Selector7/1, Bus Selector/1, Bus Selector3/1
  Bus Selector7/2 -> Sum1/1  "<cmd_q2_dd>"
  Sum/1 -> Mux5/1
  C_q2/1 -> Sum1/2  "Tm2"
  Sum1/1 -> Mux5/2
  [PLANT] -> Bus Selector4/1
  Bus Selector4/1 -> Mux7/1  "<q1_d>"
  Bus Selector4/2 -> Mux7/2  "<q2_d>"
  Mux7/1 -> Reshape5/1
  Reshape5/1 -> Product2/2  "q_d"
  Sum2/1 -> Scope1/1, Product1/2  "y"
  Bus Selector7/1 -> Sum/1  "<cmd_q1_dd>"
  Gain1/1 -> simplified_model/2(L_1y)
  Gain2/1 -> Gravity compensation/2(L_2x), simplified_model/3(L_2x)
  Gain9/1 -> simplified_model/4(L_2y)
  Gain10/1 -> simplified_model/5(b1)
  Gain11/1 -> simplified_model/6(b2)
  Gain12/1 -> Gravity compensation/4(m1), simplified_model/7(m1)
  Gain14/1 -> Gravity compensation/5(m2), simplified_model/8(m2)
  Bus Selector6/1 -> Minus/1  "<cmd_q1>"
  Bus Selector8/1 -> Minus/2  "<q1>"
  [CMD] -> Bus Selector6/1
  [PLANT] -> Bus Selector8/1
  [PLANT] -> Bus Selector10/1
  Bus Selector9/1 -> Minus1/1  "<cmd_q2>"
  Bus Selector10/1 -> Minus1/2  "<q2>"
  [CMD] -> Bus Selector9/1
  Bus Selector13/1 -> Minus2/2  "<q1_d>"
  [CMD] -> Bus Selector12/1
  Bus Selector11/1 -> Minus3/2  "<q2_d>"
  Bus Selector12/1 -> Minus2/1  "<cmd_q1_d>"
  [CMD] -> Bus Selector14/1
  Bus Selector14/1 -> Minus3/1  "<cmd_q2_d>"
  [PLANT] -> Bus Selector13/1
  [PLANT] -> Bus Selector11/1
  Mux1/1 -> Reshape3/1
  Minus/1 -> Mux3/1
  Minus1/1 -> Mux3/2
  Mux3/1 -> Mux1/1  "delta_q"
  Minus3/1 -> Mux4/2
  Minus2/1 -> Mux4/1
  Mux4/1 -> Mux1/2  "delta_q_d"
  Reshape3/1 -> Matrix Multiply/2  "y"
  Constant1/1 -> Matrix Multiply/1
  Matrix Multiply/1 -> Scope5/1, Matrix 1-Norm/1, MATLAB Function/1(z)  "z"
  MATLAB Function/1(w) -> Sum2/2, Scope/1  "w"
  Reshape1/1 -> Sum2/1
  Constant4/1 -> MATLAB Function/2(epsilon)
  Constant3/1 -> MATLAB Function/3(rho)
  Matrix 1-Norm/1 -> Scope4/1
  Zero-Order Hold2/1 -> [CMD]
  Zero-Order Hold1/1 -> [PLANT]
  Zero-Order Hold3/1 -> tau/1
  Constant17/1 -> Gravity compensation/3(g)
  Gain3/1 -> Gravity compensation/1(L_1x), simplified_model/1(L_1x)
  simplified_model/1(M_bar) -> Product1/1
  Product2/1 -> Sum3/2
  Product1/1 -> Sum3/1
  simplified_model/2(Fv) -> Product2/1
  Gravity compensation/1(G) -> Sum3/3

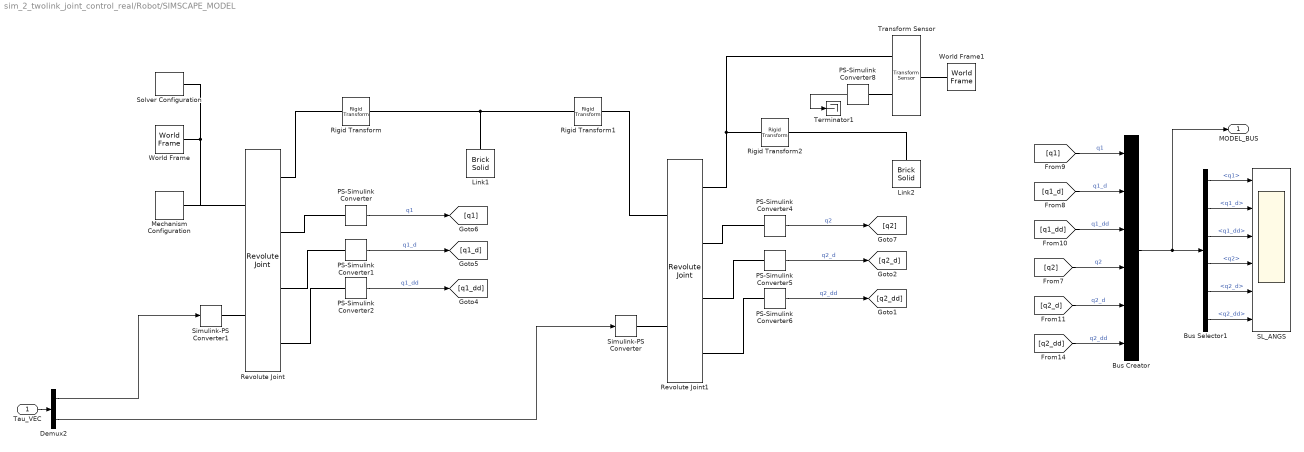
== system sim_2_twolink_joint_control_real/Robot/SIMSCAPE_MODEL ==
  Tau_VEC : Inport
  Bus Creator : BusCreator  Inputs=6
  Bus Selector1 : BusSelector  OutputSignals=q1,q1_d,q1_dd,q2,q2_d,q2_dd
  Demux2 : Demux  Outputs=2
  Link1 : sm_lib/Body Elements/Brick Solid  GraphicAmbientColor=[0.15 0.15 0.15 1.0]  BasedOnType=Density  BrickDimensions=[L1x L1y L1z]  BrickDimensionUnits=m  CenterOfMass=[0 0 0]  CenterOfMassUnits=m  GraphicDiffuseColor=[0.8 0.8 1.0]  Density=density  DensityUnits=kg/m^3  DoExposeReferenceFrame=on  GraphicEmissiveColor=[0.0 0.0 0.0 1.0]  ExportEntireGeometry=off  SerializedFrames=<Frames/>  MarkerShape=Sphere  MarkerSize=10  GraphicType=FromGeometry  InertiaType=CalculateFromGeometry  Mass=1  MassUnits=kg  MomentsOfInertia=[1 1 1]  MomentsOfInertiaUnits=kg*m^2  GraphicOpacity=1.0  ProductsOfInertia=[0 0 0]  ProductsOfInertiaUnits=kg*m^2  GraphicShininess=75  GraphicSpecularColor=[0.5 0.5 0.5 1.0]  GraphicVisPropType=SimpleVisualProperties
  Link2 : sm_lib/Body Elements/Brick Solid  GraphicAmbientColor=[0.15 0.15 0.15 1.0]  BasedOnType=Density  BrickDimensions=[L2x L2y L2z]  BrickDimensionUnits=m  CenterOfMass=[0 0 0]  CenterOfMassUnits=m  GraphicDiffuseColor=[1.0 0.6 1.0]  Density=density  DensityUnits=kg/m^3  DoExposeReferenceFrame=on  GraphicEmissiveColor=[0.0 0.0 0.0 1.0]  ExportEntireGeometry=off  SerializedFrames=<Frames/>  MarkerShape=Sphere  MarkerSize=10  GraphicType=FromGeometry  InertiaType=CalculateFromGeometry  Mass=1  MassUnits=kg  MomentsOfInertia=[1 1 1]  MomentsOfInertiaUnits=kg*m^2  GraphicOpacity=1.0  ProductsOfInertia=[0 0 0]  ProductsOfInertiaUnits=kg*m^2  GraphicShininess=75  GraphicSpecularColor=[0.5 0.5 0.5 1.0]  GraphicVisPropType=SimpleVisualProperties
  Mechanism Configuration : sm_lib/Utilities/Mechanism Configuration  UniformGravity=Constant  GravityVector=[0 -g 0 ]  GravityVectorUnits=m/s^2  GravityUnits=m/s^2  LinearizationDelta=1e-4  JointModeTransitionNonlinearIterations=2
  PS-Simulink Converter : nesl_utility/PS-Simulink Converter  PhysicalDomain=network_engine_domain  SubClassName=ps_output  LeftPortType=input  RightPortType=output  PseudoPeriodic=off  Frequencies=[]  Unit=rad  AffineConversion=off
      settings: SourceProductBaseCode=PW,SS
  PS-Simulink Converter1 : nesl_utility/PS-Simulink Converter  PhysicalDomain=network_engine_domain  SubClassName=ps_output  LeftPortType=input  RightPortType=output  PseudoPeriodic=off  Frequencies=[]  Unit=rad/s  AffineConversion=off
      settings: SourceProductBaseCode=PW,SS
  PS-Simulink Converter2 : nesl_utility/PS-Simulink Converter  PhysicalDomain=network_engine_domain  SubClassName=ps_output  LeftPortType=input  RightPortType=output  PseudoPeriodic=off  Frequencies=[]  Unit=rad/s^2  AffineConversion=off
      settings: SourceProductBaseCode=PW,SS
  PS-Simulink Converter4 : nesl_utility/PS-Simulink Converter  PhysicalDomain=network_engine_domain  SubClassName=ps_output  LeftPortType=input  RightPortType=output  PseudoPeriodic=off  Frequencies=[]  Unit=rad  AffineConversion=off
      settings: SourceProductBaseCode=PW,SS
  PS-Simulink Converter5 : nesl_utility/PS-Simulink Converter  PhysicalDomain=network_engine_domain  SubClassName=ps_output  LeftPortType=input  RightPortType=output  PseudoPeriodic=off  Frequencies=[]  Unit=rad/s  AffineConversion=off
      settings: SourceProductBaseCode=PW,SS
  PS-Simulink Converter6 : nesl_utility/PS-Simulink Converter  PhysicalDomain=network_engine_domain  SubClassName=ps_output  LeftPortType=input  RightPortType=output  PseudoPeriodic=off  Frequencies=[]  Unit=rad/s^2  AffineConversion=off
      settings: SourceProductBaseCode=PW,SS
  PS-Simulink Converter8 : nesl_utility/PS-Simulink Converter  PhysicalDomain=network_engine_domain  SubClassName=ps_output  LeftPortType=input  RightPortType=output  PseudoPeriodic=off  Frequencies=[]  Unit=1  AffineConversion=off
      settings: SourceProductBaseCode=PW,SS
  Revolute Joint : sm_lib/Joints/Revolute Joint  JointMode=Normal  SenseConstraintForce=off  SenseConstraintForceX=off  SenseConstraintForceY=off  SenseConstraintForceZ=off  SenseConstraintTorque=off  SenseConstraintTorqueX=off  SenseConstraintTorqueY=off  SenseConstraintTorqueZ=off  SenseTotalForce=off  SenseTotalForceX=off  SenseTotalForceY=off  SenseTotalForceZ=off  SenseTotalTorque=off  SenseTotalTorqueX=off  SenseTotalTorqueY=off  SenseTotalTorqueZ=off  CompositeWrenchDir=BaseOnFollower  CompositeWrenchFrame=BaseFrame  EquilibriumPosition=0  EquilibriumPositionUnits=deg  SpringStiffness=0  SpringStiffnessUnits=N*m/deg  DampingCoefficient=b1  DampingCoefficientUnits=N*m/(rad/s)  TorqueActuationMode=InputTorque  MotionActuationMode=ComputedMotion  SensePosition=on  SenseVelocity=on  SenseAcceleration=on  SenseTorqueForce=off  SenseLowerLimitTorqueForce=off  SenseUpperLimitTorqueForce=off  LowerLimitSpecify=off  LowerLimitBound=-90  LowerLimitBoundUnits=deg  LowerLimitStiffness=1e4  LowerLimitStiffnessUnits=N*m/deg  LowerLimitDamping=10  LowerLimitDampingUnits=N*m/(deg/s)  LowerLimitTransitionRegionWidth=0.1  LowerLimitTransitionRegionWidthUnits=deg  UpperLimitSpecify=off  UpperLimitBound=90  UpperLimitBoundUnits=deg  UpperLimitStiffness=1e4  UpperLimitStiffnessUnits=N*m/deg  UpperLimitDamping=10  UpperLimitDampingUnits=N*m/(deg/s)  UpperLimitTransitionRegionWidth=0.1  UpperLimitTransitionRegionWidthUnits=deg  PositionTargetSpecify=on  PositionTargetPriority=Low  PositionTargetValue=theta1_0  PositionTargetValueUnits=rad  VelocityTargetSpecify=on  VelocityTargetPriority=High  VelocityTargetValue=theta1_dot_0  VelocityTargetValueUnits=rad/s
      settings: AttributesFormatString=|
      | %<DampingCoefficient>
      | %<PositionTargetValue>
      | %<VelocityTargetValue>
  Revolute Joint1 : sm_lib/Joints/Revolute Joint  JointMode=Normal  SenseConstraintForce=off  SenseConstraintForceX=off  SenseConstraintForceY=off  SenseConstraintForceZ=off  SenseConstraintTorque=off  SenseConstraintTorqueX=off  SenseConstraintTorqueY=off  SenseConstraintTorqueZ=off  SenseTotalForce=off  SenseTotalForceX=off  SenseTotalForceY=off  SenseTotalForceZ=off  SenseTotalTorque=off  SenseTotalTorqueX=off  SenseTotalTorqueY=off  SenseTotalTorqueZ=off  CompositeWrenchDir=BaseOnFollower  CompositeWrenchFrame=FollowerFrame  EquilibriumPosition=0  EquilibriumPositionUnits=deg  SpringStiffness=0  SpringStiffnessUnits=N*m/deg  DampingCoefficient=b2  DampingCoefficientUnits=N*m/(rad/s)  TorqueActuationMode=InputTorque  MotionActuationMode=ComputedMotion  SensePosition=on  SenseVelocity=on  SenseAcceleration=on  SenseTorqueForce=off  SenseLowerLimitTorqueForce=off  SenseUpperLimitTorqueForce=off  LowerLimitSpecify=off  LowerLimitBound=-90  LowerLimitBoundUnits=deg  LowerLimitStiffness=1e4  LowerLimitStiffnessUnits=N*m/deg  LowerLimitDamping=10  LowerLimitDampingUnits=N*m/(deg/s)  LowerLimitTransitionRegionWidth=0.1  LowerLimitTransitionRegionWidthUnits=deg  UpperLimitSpecify=off  UpperLimitBound=90  UpperLimitBoundUnits=deg  UpperLimitStiffness=1e4  UpperLimitStiffnessUnits=N*m/deg  UpperLimitDamping=10  UpperLimitDampingUnits=N*m/(deg/s)  UpperLimitTransitionRegionWidth=0.1  UpperLimitTransitionRegionWidthUnits=deg  PositionTargetSpecify=on  PositionTargetPriority=Low  PositionTargetValue=theta2_0  PositionTargetValueUnits=rad  VelocityTargetSpecify=on  VelocityTargetPriority=High  VelocityTargetValue=theta2_dot_0  VelocityTargetValueUnits=rad/s
      settings: AttributesFormatString=|
      | %<DampingCoefficient>
      | %<PositionTargetValue>
      | %<VelocityTargetValue>
  Rigid Transform : sm_lib/Frames and Transforms/Rigid Transform  TranslationMethod=StandardAxis  TranslationStandardOffset=L1x/2  TranslationLengthUnit=m  TranslationStandardAxis=+X  TranslationCartesianOffset=[0 0 0]  TranslationROffset=0  TranslationROffsetUnits=m  TranslationZOffset=0  TranslationZOffsetUnits=m  TranslationThetaOffset=0  TranslationThetaOffsetUnits=deg  RotationMethod=None  RotationAngleUnits=deg  RotationStandardAxis=+Z  RotationAngle=0.0  RotationArbitraryAxis=[0 0 1]  FollAlignAxisA=+X  BaseAlignAxisA=+Y  FollAlignAxisB=+Y  BaseAlignAxisB=+Z  RotationSequenceAxes=FollowerAxes  RotationSequence=XYX  RotationSequenceAngles=[0 0 0]  RotationSequenceAnglesUnits=deg  RotationMatrix=[1 0 0; 0 1 0; 0 0 1]
  Rigid Transform1 : sm_lib/Frames and Transforms/Rigid Transform  TranslationMethod=StandardAxis  TranslationStandardOffset=L1x/2  TranslationLengthUnit=m  TranslationStandardAxis=+X  TranslationCartesianOffset=[0 0 0]  TranslationROffset=0  TranslationROffsetUnits=m  TranslationZOffset=0  TranslationZOffsetUnits=m  TranslationThetaOffset=0  TranslationThetaOffsetUnits=deg  RotationMethod=None  RotationAngleUnits=deg  RotationStandardAxis=+Z  RotationAngle=0.0  RotationArbitraryAxis=[0 0 1]  FollAlignAxisA=+X  BaseAlignAxisA=+Y  FollAlignAxisB=+Y  BaseAlignAxisB=+Z  RotationSequenceAxes=FollowerAxes  RotationSequence=XYX  RotationSequenceAngles=[0 0 0]  RotationSequenceAnglesUnits=deg  RotationMatrix=[1 0 0; 0 1 0; 0 0 1]
  Rigid Transform2 : sm_lib/Frames and Transforms/Rigid Transform  TranslationMethod=StandardAxis  TranslationStandardOffset=L2x/2  TranslationLengthUnit=m  TranslationStandardAxis=+X  TranslationCartesianOffset=[0 0 0]  TranslationROffset=0  TranslationROffsetUnits=m  TranslationZOffset=0  TranslationZOffsetUnits=m  TranslationThetaOffset=0  TranslationThetaOffsetUnits=deg  RotationMethod=None  RotationAngleUnits=deg  RotationStandardAxis=+Z  RotationAngle=0.0  RotationArbitraryAxis=[0 0 1]  FollAlignAxisA=+X  BaseAlignAxisA=+Y  FollAlignAxisB=+Y  BaseAlignAxisB=+Z  RotationSequenceAxes=FollowerAxes  RotationSequence=XYX  RotationSequenceAngles=[0 0 0]  RotationSequenceAnglesUnits=deg  RotationMatrix=[1 0 0; 0 1 0; 0 0 1]
  SL_ANGS : Scope  NumInputPorts=6
  Simulink-PS Converter : nesl_utility/Simulink-PS Converter  PhysicalDomain=network_engine_domain  SubClassName=ps_input  LeftPortType=input  RightPortType=output  PseudoPeriodic=off  Frequencies=[]  NoiseDistribution=none  NoiseParameters=[]  Unit=N*m  AffineConversion=off  FilteringAndDerivatives=zero  SimscapeFilterOrder=1  InputFilterTimeConstant=0.001  UdotUserProvided=1
      settings: SourceProductBaseCode=PW,SS
  Simulink-PS Converter1 : nesl_utility/Simulink-PS Converter  PhysicalDomain=network_engine_domain  SubClassName=ps_input  LeftPortType=input  RightPortType=output  PseudoPeriodic=off  Frequencies=[]  NoiseDistribution=none  NoiseParameters=[]  Unit=N*m  AffineConversion=off  FilteringAndDerivatives=zero  SimscapeFilterOrder=1  InputFilterTimeConstant=0.001  UdotUserProvided=1
      settings: SourceProductBaseCode=PW,SS
  Solver Configuration : nesl_utility/Solver Configuration  PhysicalDomain=network_engine_domain  SubClassName=solver  LeftPortType=input  RightPortType=generic  Tones=[]  Harmonics=[]  SimulateNoise=off  Profile=off  UseLocalSampling=off  EnableSwitchedLinearOptims=on  FrequencyDomain=off  UseCCode=off  RelTol=0.001  AbsTol=1e-06  MinStep=1e-09  ToWorkspace=off  RevertToSquareIcSolve=off  NumHomotopyIterations=100  PhasorMode=off  PhasorModeNumHarmonics=1  DoDC=off  ResidualTolerance=1e-09  UseLocalSolver=off  LocalSolverChoice=NE_TRAPEZOIDAL_ADVANCER  LocalSolverSampleTime=0.01  DoFixedCost=off  MaxNonlinIter=3  MaxModeIter=2  ComputeImpulses=off  ImpulseIterations=2  LinearAlgebra=Sparse  EquationFormulation=NE_TIME_EF  DelaysMemoryBudget=1024  AutomaticFiltering=off  FilteringTimeConstant=0.001  PartitionStorageMethod=AS_NEEDED  PartitionMemoryBudget=1024  PartitionMethod=FAST
      settings: SourceProductBaseCode=PW,SS
  Terminator1 : Terminator
  Transform Sensor : sm_lib/Frames and Transforms/Transform Sensor  MeasurementFrame=World  SenseAngle=off  SenseAxis=off  SenseAngle1=off  SenseAngle2=off  SenseAngle3=off  SenseQ=off  SenseR=on  SenseOmegaX=off  SenseOmegaY=off  SenseOmegaZ=off  SenseOmega1=off  SenseOmega2=off  SenseOmega3=off  SenseQDot=off  SenseRDot=off  SenseAlphaX=off  SenseAlphaY=off  SenseAlphaZ=off  SenseAlpha1=off  SenseAlpha2=off  SenseAlpha3=off  SenseQDDot=off  SenseRDDot=off  SenseX=off  SenseY=off  SenseZ=off  SenseRad=off  SenseAzim=off  SenseDist=off  SenseInc=off  SenseXDot=off  SenseYDot=off  SenseZDot=off  SenseRadDot=off  SenseAzimDot=off  SenseDistDot=off  SenseIncDot=off  SenseXDDot=off  SenseYDDot=off  SenseZDDot=off  SenseRadDDot=off  SenseAzimDDot=off  SenseDistDDot=off  SenseIncDDot=off
  World Frame : sm_lib/Frames and Transforms/World Frame
  World Frame1 : sm_lib/Frames and Transforms/World Frame
  MODEL_BUS : Outport
  wires:
  PS-Simulink Converter/1 -> [q1]  "q1"
  PS-Simulink Converter2/1 -> [q1_dd]  "q1_dd"
  PS-Simulink Converter1/1 -> [q1_d]  "q1_d"
  Bus Creator/1 -> Bus Selector1/1, MODEL_BUS/1
  PS-Simulink Converter4/1 -> [q2]  "q2"
  PS-Simulink Converter6/1 -> [q2_dd]  "q2_dd"
  PS-Simulink Converter5/1 -> [q2_d]  "q2_d"
  Tau_VEC/1 -> Demux2/1
  Demux2/1 -> Simulink-PS Converter1/1
  Demux2/2 -> Simulink-PS Converter/1
  Bus Selector1/2 -> SL_ANGS/2  "<q1_d>"
  Bus Selector1/5 -> SL_ANGS/5  "<q2_d>"
  Bus Selector1/6 -> SL_ANGS/6  "<q2_dd>"
  Bus Selector1/1 -> SL_ANGS/1  "<q1>"
  Bus Selector1/3 -> SL_ANGS/3  "<q1_dd>"
  [q1_dd] -> Bus Creator/3  "q1_dd"
  [q1] -> Bus Creator/1  "q1"
  [q2] -> Bus Creator/4  "q2"
  [q2_d] -> Bus Creator/5  "q2_d"
  [q1_d] -> Bus Creator/2  "q1_d"
  [q2_dd] -> Bus Creator/6  "q2_dd"
  Bus Selector1/4 -> SL_ANGS/4  "<q2>"
  PS-Simulink Converter8/1 -> Terminator1/1
  connections:
  World Frame/RConn1 -- Revolute Joint/LConn1 -- Mechanism Configuration/RConn1 -- Solver Configuration/RConn1
  Rigid Transform1/LConn1 -- Link1/RConn1 -- Rigid Transform/RConn1
  Revolute Joint/RConn3 -- PS-Simulink Converter1/LConn1
  Revolute Joint/RConn4 -- PS-Simulink Converter2/LConn1
  Rigid Transform/LConn1 -- Revolute Joint/RConn1
  PS-Simulink Converter/LConn1 -- Revolute Joint/RConn2
  Revolute Joint1/LConn1 -- Rigid Transform1/RConn1
  Revolute Joint1/RConn3 -- PS-Simulink Converter5/LConn1
  Revolute Joint1/RConn2 -- PS-Simulink Converter4/LConn1
  Revolute Joint1/RConn4 -- PS-Simulink Converter6/LConn1
  Link2/RConn1 -- Rigid Transform2/RConn1
  Rigid Transform2/LConn1 -- Transform Sensor/RConn1 -- Revolute Joint1/RConn1
  World Frame1/RConn1 -- Transform Sensor/LConn1
  PS-Simulink Converter8/LConn1 -- Transform Sensor/RConn2
  Simulink-PS Converter/RConn1 -- Revolute Joint1/LConn2
  Simulink-PS Converter1/RConn1 -- Revolute Joint/LConn2

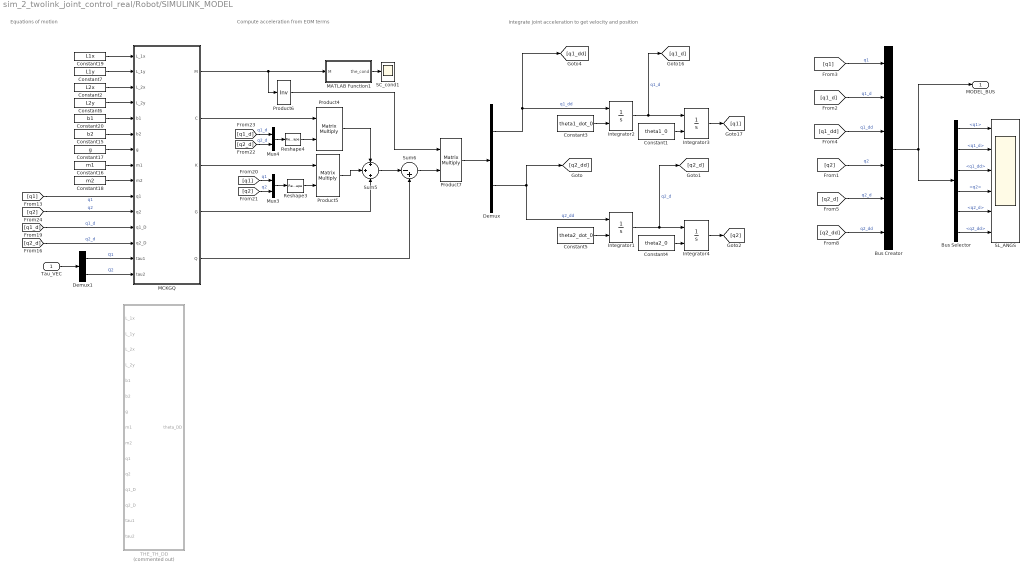
== system sim_2_twolink_joint_control_real/Robot/SIMULINK_MODEL ==
  note: Integrate joint acceleration to get velocity and position
  note: Compute acceleration from EOM terms
  note: Equations of motion
  Tau_VEC : Inport
  Bus Creator : BusCreator  Inputs=6
  Bus Selector : BusSelector  OutputSignals=q1,q1_d,q1_dd,q2,q2_d,q2_dd
  Constant1 : Constant  Value=theta1_0
  Constant15 : Constant  Value=b2
  Constant16 : Constant  Value=m1
  Constant17 : Constant  Value=g
  Constant18 : Constant  Value=m2
  Constant19 : Constant  Value=L1x
  Constant2 : Constant  Value=L2x
  Constant20 : Constant  Value=b1
  Constant3 : Constant  Value=theta1_dot_0
  Constant4 : Constant  Value=theta2_0
  Constant5 : Constant  Value=theta2_dot_0
  Constant6 : Constant  Value=L2y
  Constant7 : Constant  Value=L1y
  Demux : Demux  Outputs=2
  Demux1 : Demux  Outputs=2
  Integrator{1..4} (4 alike) : Integrator  InitialConditionSource=external
  MATLAB Function1 : MATLAB Function  TreatAsAtomicUnit=on
  MCKGQ : MATLAB Function  TreatAsAtomicUnit=on
  Mux3 : Mux  Inputs=2
  Mux4 : Mux  Inputs=2
  Product4 : Product  Multiplication=Matrix(*)
  Product5 : Product  Multiplication=Matrix(*)
  Product6 : Product  Inputs=/  Multiplication=Matrix(*)
  Product7 : Product  Multiplication=Matrix(*)
  Reshape3 : Reshape  OutputDimensionality=Column vector (2-D)
  Reshape4 : Reshape  OutputDimensionality=Column vector (2-D)
  SC_cond1 : Scope
  SL_ANGS : Scope  NumInputPorts=6
  Sum5 : Sum  Inputs=+|+|+
  Sum6 : Sum  Inputs=|-+
  THE_TH_DD : MATLAB Function  Commented=on  TreatAsAtomicUnit=on
  MODEL_BUS : Outport
  wires:
  Bus Creator/1 -> Bus Selector/1, MODEL_BUS/1
  Bus Selector/2 -> SL_ANGS/2  "<q1_d>"
  Bus Selector/3 -> SL_ANGS/3  "<q1_dd>"
  Bus Selector/1 -> SL_ANGS/1  "<q1>"
  Bus Selector/4 -> SL_ANGS/4  "<q2>"
  Bus Selector/6 -> SL_ANGS/6  "<q2_dd>"
  Integrator3/1 -> [q1]
  Integrator2/1 -> [q1_d], Integrator3/1  "q1_d"
  Constant3/1 -> Integrator2/2
  Constant1/1 -> Integrator3/2
  Integrator1/1 -> [q2_d], Integrator4/1  "q2_d"
  Constant4/1 -> Integrator4/2
  Integrator4/1 -> [q2]
  Constant5/1 -> Integrator1/2
  [q1_d] -> Bus Creator/2  "q1_d"
  [q2_d] -> Bus Creator/5  "q2_d"
  [q2] -> Bus Creator/4  "q2"
  [q2_dd] -> Bus Creator/6  "q2_dd"
  [q1] -> Bus Creator/1  "q1"
  [q1_dd] -> Bus Creator/3  "q1_dd"
  Demux/1 -> [q1_dd], Integrator2/1  "q1_dd"
  Demux/2 -> [q2_dd], Integrator1/1  "q2_dd"
  MCKGQ/5(Q) -> Sum6/2
  [q1] -> Mux3/1  "q1"
  Sum6/1 -> Product7/2
  [q2] -> Mux3/2  "q2"
  Sum5/1 -> Sum6/1
  Product4/1 -> Sum5/1
  Constant18/1 -> MCKGQ/9(m2)
  Product5/1 -> Sum5/2
  Demux1/2 -> MCKGQ/15(tau2)  "Q2"
  MCKGQ/3(K) -> Product5/1
  MATLAB Function1/1(the_cond) -> SC_cond1/1
  Product6/1 -> Product7/1
  Constant20/1 -> MCKGQ/5(b1)
  Reshape3/1 -> Product5/2
  [q1] -> MCKGQ/10(q1)  "q1"
  Constant6/1 -> MCKGQ/4(L_2y)
  MCKGQ/4(G) -> Sum5/3
  Constant15/1 -> MCKGQ/6(b2)
  [q1_d] -> MCKGQ/12(q1_D)  "q1_d"
  Constant2/1 -> MCKGQ/3(L_2x)
  Constant19/1 -> MCKGQ/1(L_1x)
  Constant7/1 -> MCKGQ/2(L_1y)
  MCKGQ/2(C) -> Product4/1
  [q1_d] -> Mux4/1  "q1_d"
  Mux3/1 -> Reshape3/1
  Reshape4/1 -> Product4/2
  [q2_d] -> MCKGQ/13(q2_D)  "q2_d"
  [q2_d] -> Mux4/2  "q2_d"
  Demux1/1 -> MCKGQ/14(tau1)  "Q1"
  MCKGQ/1(M) -> MATLAB Function1/1(M), Product6/1
  Mux4/1 -> Reshape4/1
  [q2] -> MCKGQ/11(q2)  "q2"
  Constant17/1 -> MCKGQ/7(g)
  Constant16/1 -> MCKGQ/8(m1)
  Tau_VEC/1 -> Demux1/1
  Product7/1 -> Demux/1
  Bus Selector/5 -> SL_ANGS/5  "<q2_d>"

== system sim_2_twolink_joint_control_real/Torqu limit/limited_torque ==
  In1 : Inport
  Demux : Demux  Outputs=2
  Mux1 : Mux  Inputs=2
  tau1_limit : Saturate  UpperLimit=max_joint_torque1  LowerLimit=-max_joint_torque1
  tau2_limit : Saturate  UpperLimit=max_joint_torque2  LowerLimit=-max_joint_torque2
  Out1 : Outport
  wires:
  tau2_limit/1 -> Mux1/2
  Mux1/1 -> Out1/1
  tau1_limit/1 -> Mux1/1
  In1/1 -> Demux/1
  Demux/1 -> tau1_limit/1
  Demux/2 -> tau2_limit/1
